simulink model "kArNa"  (R2024a)
settings: Solver=ode15s  StartTime=0.0  StopTime=721  FixedStep=0.01  MaxStep=0.5  RelTol=1e-5
PreLoadFcn:
  | %% Load parameter values:
  | 
  | load('solardata')
  | load('matincl')
  | load('trackdata3')
  | 
  | %% Parameter structures -------------------------------
  | panel = struct();
  | pipe = struct();
  | tank = struct();
  | pumps = struct();
  | 
  | %% Load parameters ------------------------------------
  | 
  | load.R = 4.5;  %Resistance. With default parameters, 4.5 Ohm is approximately optimal for maximum electrical power extraction
  | 
  | 
  | %% Solar panel parameters ------------------------------
  | 
  | % Initial temperatures [K]
  | panel.initial.Tg0 = 295; %Glass cover
  | panel.initial.Tpv0 = 295; %PV cells
  | panel.initial.Te0 = 295; %Heat exchanger
  | panel.initial.Tw0 = 295; %Water in the tank
  | panel.initial.Tb0 = 295; %Back cover
  | 
  | % Geometry
  | panel.geometry.Acell = 0.0225; %Area of a cell, [m^2]
  | panel.geometry.Ncell = 72; %Number of cells
  | 
  | % Optical properties
  | panel.optical.ng = 1.52; %Refractive index ratio glass/air
  | panel.optical.absg = 0.2; %Absorption coefficient of glass per unit length [1/m]
  | panel.optical.dg = 0.01; %Thickness of glass cover [m]
  | panel.optical.rpv = 0.15; %Reflection factor of PV cell
  | 
  | % Heat transfer properties
  | panel.heatTransfer.Ta = 295;  %Temperature of ambient air [K]
  | panel.heatTransfer.Tsky = 290;%Temperature of sky (for radiative heat transfer) [K]
  | 
  | panel.heatTransfer.Mg = 4; %Mass of glass cover [kg]
  | panel.heatTransfer.Mpv = 0.2; %Mass of one PV cell [kg]
  | panel.heatTransfer.Me = 15; %Mass of heat exchanger [kg]
  | panel.heatTransfer.Mb = 5; %Mass of back cover [kg]
  | 
  | panel.heatTransfer.Cg = 800; %Specific heat of glass [J/kg/K]
  | panel.heatTransfer.Cpv = 200; %Specific heat of PV cell [J/kg/K]
  | panel.heatTransfer.Ce = 460; %Specific heat of heat exchanger [J/kg/K]
  | panel.heatTransfer.Cb = 400; %Specific heat of back cover [J/kg/K]
  | 
  | panel.heatTransfer.epsg = 0.75; %Emissivity of glass
  | panel.heatTransfer.epspv = 0.7; %Emissivity of PV cell
  | 
  | panel.heatTransfer.hga = 10;%Free convection coefficient between glass and ambient air [W/m^2/K]
  | panel.heatTransfer.hgpv = 20; %Free convection coefficient between PV cells and glass [W/m^2/K]
  | panel.heatTransfer.hba = 10;%Free convection coefficient between back cover and ambient air [W/m^2/K]
  | 
  | panel.heatTransfer.ke = 130;%Thermal conductivity of heat exchanger [W/m/K]
  | panel.heatTransfer.Le = 0.04;%Thickness of heat exchanger [m]
  | panel.heatTransfer.kins = 0.1;%Thermal conductivity of insulation layer [W/m/K]
  | panel.heatTransfer.Lins = 0.03;%Thickness of insulation layer [m]
  | 
  | % PV cell electrical properties
  | panel.pv.Isc = 8.88; % Short-circuit current, Isc [A]
  | panel.pv.Voc = 0.62;% Open-circuit voltage, Voc [V]
  | panel.pv.Is  = 1e-6; % Diode saturation current, Is [A]
  | panel.pv.Is2 = 0; % Diode saturation current, Is2 [A]
  | panel.pv.Iph0 = 8.88;% Solar-generated current for measurements, Iph0 [A]
  | panel.pv.Ir0 = 1000;% Irradiance used for measurements, Ir0 [W/m^2]
  | panel.pv.ec = 1.5; % Quality factor, N
  | panel.pv.N2 = 2; % Quality factor, N2
  | panel.pv.Rs = 0;  % Series resistance, Rs [Ohm]
  | panel.pv.Rp = inf ; % Parallel resistance, Rp [Ohm]
  | panel.pv.TIPH1 = 0; % First order temperature coefficient for Iph, TIPH1 [1/K]
  | panel.pv.EG  = 1.11;% Energy gap, EG [eV]
  | panel.pv.TXIS1 = 3;% Temperature exponent for Is, TXIS1
  | panel.pv.TXIS2 = 3;% Temperature exponent for Is2, TXIS2
  | panel.pv.TRS1 = 0;% Temperature exponent for Rs, TRS1
  | panel.pv.TRP1 = 0;% Temperature exponent for Rp, TRP1
  | panel.pv.Tmeas = 25; % Measurement temperature [degC]
model workspace: external: MATLAB File sm_solar_tracker_parameters.m (data not in the file)
values from neighbouring files (symbols this model uses):
  matincl = [1.57079632679 1.57079632679 1.57079632679 1.57079632679 1.57079632679 1.57079632679 1.57079632679 1.57079632679 1.57079632679 1.57079632679 1.57079632679 1.57079632679 ... (721 elements, 1x721)]    [matincl.mat]
  solardata = [0 0 0 0 0 0 0 0 0 0 0 0 ... (721 elements, 1x721)]    [solardata.mat]
  trackdata3 = [3.66156931996e-23 3.03330898688e-07 9.13986174438e-07 1.77569311168e-06 2.76980746682e-06 3.72542605559e-06 4.44246757577e-06 4.72588119878e-06 4.72601258328e-06 4.79496576622e-06 5.00722746548e-06 5.38898182365e-06 ... (721 elements, 1x721)]    [trackdata3.mat]
undefined symbols (not defined in the file or in its folder): X, Y, Z
libraries: fl_lib x14, nesl_utility x11, WormAndGearConstraintLibrary x6, sm_lib x4, ee_lib x2, dspsigops x1
CloseFcn:
  | %% Close figures
  | try, close(figHandlePumpInputs), end;
  | try, close(figHandleSolarInputs), end;
  | try, close(figHandleOptics), end;
  | try, close(figHandleOutputs), end;
  | 
  | clear load
  | clear panel
  | clear pipe
  | clear pumps
  | clear tank
  | 
  | clear Absg angle demand_t demand_y E_elec E_input E_therm E_therm_source;
  | clear figHandleOptics figHandleOutputs figHandlePumpInputs figHandleSolarInputs;
  | clear internal_flow_t internal_flow_y model out Pow_elec_series Pow_input_series;
  | clear Pow_therm_series Pow_therm_source_series Reflg solar_inclination_series;
  | clear solar_inclination_t solar_inclination_y solar_irradiance_series;
  | clear solar_irradiance_t solar_irradiance_y stptime supply_t supply_y;
  | clear Tb_series Te_series Tg_series tout Tpv_series Transg Tw_series Voltank_series;
  | clear absg dg ng nga r1 r1p r1s r2 r2p r2s t1 t2 taug th2
Description:
  | Using the Worm and Gear Constraint Block - Solar Tracker
  | 
  | 
  | Copyright 2008-2019 The MathWorks, Inc.
settings Model: Creator=MathWorks  LastModifiedBy=manik
settings SolverCC: AlgebraicLoopSolver=TrustRegion
settings DataIOCC: ReturnWorkspaceOutputs=off
settings DebuggingCC: UnconnectedInputMsg=warning  UnconnectedOutputMsg=warning  UnconnectedLineMsg=warning  ArithmeticOperatorsInVariantConditions=warning
settings ModelReferenceCC: EnableRefExpFcnMdlSchedulingChecks=on
settings SFSimCC: SimUseLocalCustomCode=off  CustomCodeUndefinedFunction=UseInterfaceOnly
settings RTWCC: RTWUseLocalCustomCode=off  GPUComputeCapability=3.5
settings CodeAppCC: StateflowObjectComments=on
settings ConfigComp: CovMetricSettings=dswe
settings SimscapeCC: SimscapeNormalizeSystem=off  SimscapeNominalValues="[{\"value\":\"10\",\"unit\":\"V\"},{\"value\":\"1\",\"unit\":\"A\"},{\"value\":\"10\",\"unit\":\"N*m\"},{\"value\":\"10\",\"unit\":\"bar\"},{\"value\":\"100\",\"unit\":\"kJ/kg\"},{\"value\":\"1\",\"unit\":\"kW\"},{\"value\":\"300\",\"unit\":\"K\"},{\"value\":\"100\",\"unit\":\"cm^3/s\"},{\"value\":\"1\",\"unit\":\"kN\"},{\"value\":\"1\",\"unit\":\"g/cm^3\"},{\"value\":\"1\",\"unit\":\"l\"},{\"value\":\"1\",\"unit\":\"cm^2\"},{\"value\":\"60\",\"unit\":\"Hz\"}]"  SimscapeLogType=all  SimscapeLogSimulationStatistics=on  SimscapeLogName=simlog_sm_solar_tracker
settings DiagnosticsConfigSet: SimMechanicsUnconnectedFramePorts=none
settings ExplorerConfigSet: InternalSimMechanicsExplorerSettings="<ExplorerConfiguration><canonicalview>default</canonicalview><AnimationSetting><BasePlaybackSpeed>1.0</BasePlaybackSpeed><PlaybackSpeedFactor>256.0</PlaybackSpeedFactor></AnimationSetting><TilePanel><TileInfo><Tiles Columns=\"2\" Count=\"4\" Rows=\"2\"><Column Weight=\"0.4991\"/><Column Weight=\"0.5009\"/><Row Weight=\"0.5\"/><Row Weight=\"0.5\"/><Tile Height=\"1\" Width=\"1\" X=\"0\" Y=\"0\"/><Tile Height=\"1\" Width=\"1\" X=\"0\" Y=\"1\"/><Tile Height=\"1\" Width=\"1\" X=\"1\" Y=\"0\"/><Tile Height=\"1\" Width=\"1\" X=\"1\" Y=\"1\"/></Tiles></TileInfo><SceneInfo><SceneViewer><BGColor><R>0.60000002384185791</R><G>0.60000002384185791</G><B>0.60000002384185791</B></BGColor><Camera><DoPerspective>off</DoPerspective><Position><X>-1.59395585619392932e-09</X><Y>-1.37838790385234322</Y><Z>0.873406468711440231</Z></Position><Center><X>-1.59395585619392932e-09</X><Y>0.0359901942601611458</Y><Z>0.873406468711440231</Z></Center><Up><X>0</X><Y>-0</Y><Z>1</Z></Up><ViewLimDist>1</ViewLimDist><YLim>0.899608663916587892</YLim><XLim>1.56307005355507145</XLim></Camera></SceneViewer><SceneViewer><BGColor><R>0.60000002384185791</R><G>0.60000002384185791</G><B>0.60000002384185791</B></BGColor><Camera><DoPerspective>off</DoPerspective><Position><X>-1.59395585619392932e-09</X><Y>0.0359901942601611458</Y><Z>2.41334542087606918</Z></Position><Center><X>-1.59395585619392932e-09</X><Y>0.0359901942601611458</Y><Z>0.873406455926843073</Z></Center><Up><X>0</X><Y>1</Y><Z>-0</Z></Up><ViewLimDist>1</ViewLimDist><YLim>0.296402877697841738</YLim><XLim>0.515000000000000013</XLim></Camera></SceneViewer><SceneViewer><BGColor><R>0.60000002384185791</R><G>0.60000002384185791</G><B>0.60000002384185791</B></BGColor><Camera><DoPerspective>off</DoPerspective><Position><X>1.27256003059215272</X><Y>0.0359901942601611458</Y><Z>0.87340646871144012</Z></Position><Center><X>-1.59395585619392932e-09</X><Y>0.0359901942601611458</Y><Z>0.87340646871144012</Z></Center><Up><X>-0</X><Y>0</Y><Z>1</Z></Up><ViewLimDist>1</ViewLimDist><YLim>0.899608663916587892</YLim><XLim>1.56869260770454999</XLim></Camera></SceneViewer><SceneViewer><BGColor><R>0.60000002384185791</R><G>0.60000002384185791</G><B>0.60000002384185791</B></BGColor><Camera><DoPerspective>off</DoPerspective><Position><X>0.866331353225705314</X><Y>-0.741331845233251241</Y><Z>1.79757748242861348</Z></Position><Center><X>0.0384713109530606112</X><Y>0.0865281970393926292</Y><Z>0.969717440155970056</Z></Center><Up><X>-0.408248290463863073</X><Y>0.408248290463863073</Y><Z>0.816496580927726145</Z></Up><ViewLimDist>1</ViewLimDist><YLim>0.91983101725578309</YLim><XLim>1.60395533633977161</XLim></Camera></SceneViewer></SceneInfo></TilePanel><MechEditorPanel><Cameras><Camera><Id>Camera1</Id><Value><Name>Slew Drive View</Name><NativeCamera><PositionKeyframeSet><Keyframe><Time>0</Time><Value><X>0.052898448769590822</X><Y>3.2815089600888423</Y><Z>1.0106868675116196</Z></Value></Keyframe></PositionKeyframeSet><CenterKeyframeSet><Keyframe><Time>0</Time><Value><X>-0.01109217435380673</X><Y>3.0487464713239714</Y><Z>0.94979470185928261</Z></Value></Keyframe></CenterKeyframeSet><UpVectorKeyframeSet><Keyframe><Time>0</Time><Value><X>-0.054323829999052796</X><Y>-0.23871114009518463</Y><Z>0.96956996296744424</Z></Value></Keyframe></UpVectorKeyframeSet></NativeCamera></Value></Camera></Cameras><GfxPanelCameraMap/><VideoCreator><PlaybackSpeedRatio>1.0</PlaybackSpeedRatio><FrameRate>30</FrameRate><VideoFormat>Motion JPEG AVI</VideoFormat><FrameSize>auto</FrameSize></VideoCreator></MechEditorPanel></ExplorerConfiguration>"

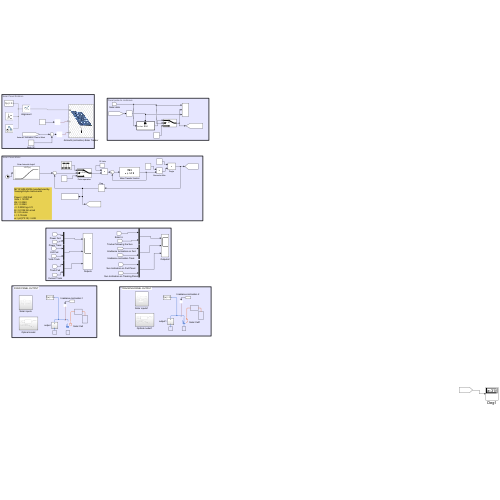
[thumbnail: Simulink's stored preview of the top-level diagram]
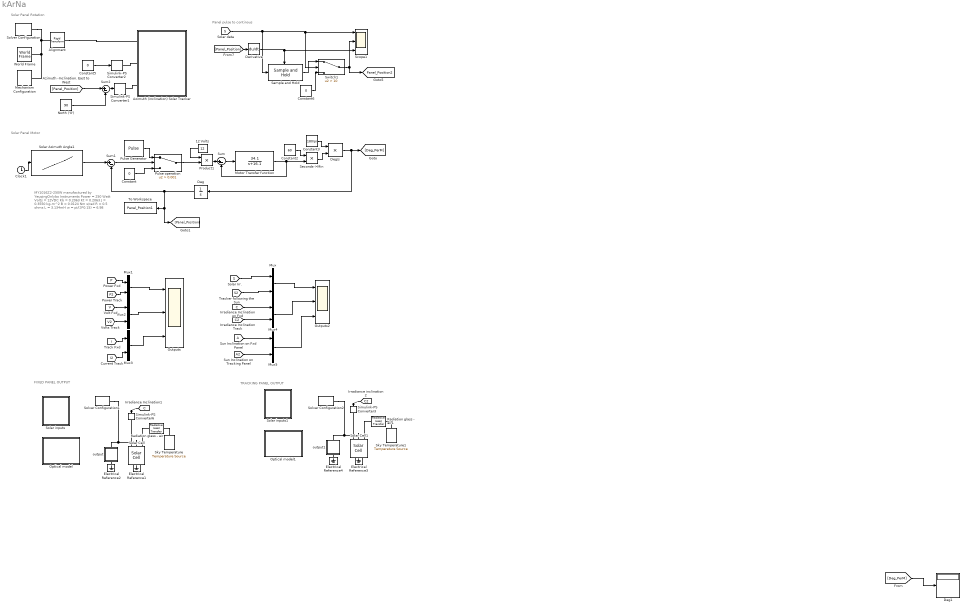
== system kArNa ==
  note: Solar Panel Motor
  note: Panel pulse to continous
  note: Solar Panel Rotation
  note: TRACKING PANEL OUTPUT
  note: FIXED PANEL OUTPUT
  note: MY1016Z2-250W manufactured by YeuqingOnlybo Instruments
      |
      | Power = 250 Watt
      | Volts = 12VDC
      | Kb = 0.2063
      | Kt = 0.2063
      | J = 0.3550 kg-m^2
      | B = 0.0124 Nm s/rad
      | R = 0.5 ohms
      | L = 3.134mH
      | w = pi/(3*0.15) = 6.98
  12 Volts : Constant  Value=12
  Alignment : sm_lib/Frames and Transforms/Rigid Transform  RotationMethod=None  FollAlignAxisA=+Z  BaseAlignAxisA=+Z  FollAlignAxisB=+Y  BaseAlignAxisB=-X  RotationStandardAxis=+Z  RotationAngle=90  RotationAngleUnits=deg  RotationArbitraryAxis=[0 0 1]  RotationSequenceAxes=FollowerAxes  RotationSequence=XYX  RotationSequenceAngles=[0 -20 0]  RotationSequenceAnglesUnits=deg  RotationMatrix=[1 0 0; 0 1 0; 0 0 1]  Quaternion=[1 0 0 0]  TranslationMethod=None  TranslationCartesianOffset=[0 0 0]  TranslationCartesianOffsetUnits=m  TranslationStandardAxis=+Z  TranslationStandardOffset=0  TranslationStandardOffsetUnits=m  TranslationROffset=0  TranslationROffsetUnits=m  TranslationThetaOffset=0  TranslationThetaOffsetUnits=deg  TranslationZOffset=0  TranslationZOffsetUnits=m
  Azimuth (inclination) Solar Tracker : Subsystem
      mask Display:
      | image(imread(fullfile(matlabroot,'toolbox','physmod','sm','smdemos','solar_tracker','images','sm_solar_tracker_solar_tracker.png')));
      | port_label('lconn',1,'B');
      | port_label('lconn',2,'y');
      | port_label('lconn',3,'p');
      | port_label('rconn',1,'w');
      | port_label('rconn',2,'t');
  Clock1 : Clock
  Constant : Constant  Value=0
  Constant2 : Constant  Value=60
  Constant3 : Constant  Value=180/pi
  Constant5 : Constant  Value=0
  Constant6 : Constant  Value=0
  Deg : Integrator
  Deg/s : Product
  Deg1 : Display
  Derivative : Derivative
  Electrical Reference{1..4} (4 alike) : fl_lib/Electrical/Electrical Elements/Electrical Reference
  Mechanism Configuration : sm_lib/Utilities/Mechanism Configuration  UniformGravity=Constant  GravityVector=[0 0 -9.80665]  GravityVectorUnits=m/s^2  LinearizationDelta=0.001  JointModeTransitionNonlinearIterations=2
  Motor Transfer function : TransferFcn  Numerator=34.1  Denominator=[1 16.1]
  Mux{,1..5} (6 alike) : Mux  Inputs=2
  North ('0') : Constant  Value=90
  Optical model : Subsystem
  Optical model1 : Subsystem
  Outputs : Scope  NumInputPorts=3
  Outputs2 : Scope  NumInputPorts=3
  Product1 : Product
  Pulse Generator : DiscretePulseGenerator  SampleTime=0.01
  Pulse operation : Switch  Criteria=u2 > Threshold  Threshold=0.001  SaturateOnIntegerOverflow=off  InputSameDT=off
  Radiation glass - air : fl_lib/Thermal/Thermal Elements/Radiative Heat Transfer  area=72*0.0225 m^2  rad_tr_coeff=5.670367e-8*0.75 W/(m^2*K^4)  T_specify=off  T_priority=None  T=0 K  T_nominal_specify=off  T_nominal_value=1  T_nominal_unit=K  Q_specify=off  Q_priority=None  Q=0 W  Q_nominal_specify=off  Q_nominal_value=1  Q_nominal_unit=W
      settings: InternalSimscapePortConfiguration="{\"Bottom\":[],\"Left\":[{\"id\":\"A\",\"label\":\"A\",\"type\":\"foundation.thermal.thermal\"}],\"Right\":[{\"id\":\"B\",\"label\":\"B\",\"type\":\"foundation.thermal.thermal\"}],\"Top\":[]}"
  Radiation glass - air1 : fl_lib/Thermal/Thermal Elements/Radiative Heat Transfer  area=72*0.0225 m^2  rad_tr_coeff=5.670367e-8*0.75 W/(m^2*K^4)  T_specify=off  T_priority=None  T=0 K  T_nominal_specify=off  T_nominal_value=1  T_nominal_unit=K  Q_specify=off  Q_priority=None  Q=0 W  Q_nominal_specify=off  Q_nominal_value=1  Q_nominal_unit=W
      settings: InternalSimscapePortConfiguration="{\"Bottom\":[],\"Left\":[{\"id\":\"A\",\"label\":\"A\",\"type\":\"foundation.thermal.thermal\"}],\"Right\":[{\"id\":\"B\",\"label\":\"B\",\"type\":\"foundation.thermal.thermal\"}],\"Top\":[]}"
  Sample and Hold : dspsigops/Sample and Hold  trig=Either edge  initCond=0  latchinput=on
  Scope1 : Scope  NumInputPorts=3
  Seconds->Min : Product
  Simulink-PS Converter1 : nesl_utility/Simulink-PS Converter  PhysicalDomain=network_engine_domain  SubClassName=ps_input  LeftPortType=input  RightPortType=output  PseudoPeriodic=off  Frequencies=[]  NoiseDistribution=none  NoiseParameters=[]  Unit=deg  AffineConversion=off  FilteringAndDerivatives=filter  SimscapeFilterOrder=2  InputFilterTimeConstant=0.2  UdotUserProvided=1
  Simulink-PS Converter2 : nesl_utility/Simulink-PS Converter  PhysicalDomain=network_engine_domain  SubClassName=ps_input  LeftPortType=input  RightPortType=output  PseudoPeriodic=off  Frequencies=[]  NoiseDistribution=none  NoiseParameters=[]  Unit=deg  AffineConversion=off  FilteringAndDerivatives=filter  SimscapeFilterOrder=2  InputFilterTimeConstant=0.2  UdotUserProvided=1
  Simulink-PS Converter3 : nesl_utility/Simulink-PS Converter  PhysicalDomain=network_engine_domain  SubClassName=ps_input  LeftPortType=input  RightPortType=output  PseudoPeriodic=off  Frequencies=[]  NoiseDistribution=none  NoiseParameters=[]  Unit=1  AffineConversion=off  FilteringAndDerivatives=provide  SimscapeFilterOrder=1  InputFilterTimeConstant=0.001  UdotUserProvided=0
  Simulink-PS Converter6 : nesl_utility/Simulink-PS Converter  PhysicalDomain=network_engine_domain  SubClassName=ps_input  LeftPortType=input  RightPortType=output  PseudoPeriodic=off  Frequencies=[]  NoiseDistribution=none  NoiseParameters=[]  Unit=1  AffineConversion=off  FilteringAndDerivatives=provide  SimscapeFilterOrder=1  InputFilterTimeConstant=0.001  UdotUserProvided=0
  Sky Temperature : fl_lib/Thermal/Thermal Sources/Temperature Source  temperature=290 K
  Sky Temperature1 : fl_lib/Thermal/Thermal Sources/Temperature Source  temperature=290 K
  Solar Azimuth Angle1 : Lookup_n-D  NumberOfTableDimensions=1  BreakpointsForDimension1=1:length(trackdata3)  Table=trackdata3  InternalRulePriority=Speed  RndMeth=Simplest
  Solar Cell : ee_lib/Sources/Solar Cell  prm=3  Isc=8.88 A  Voc=0.62 V  Is=1e-6 A  Is2=0 A  Iph=7.34 A  Ir0=1000 W/m^2  ec=1.5  N2=2  Rs=0 Ohm  Rp=inf Ohm  N_series=72  N_parallel=1  TIPH1=0 1/K  EG=1.11 eV  TXIS1=3  TXIS2=3  TRS1=0  TRP1=0  Tmeas=25 degC  TFIXED=25 degC  thermal_mass=0.2*200 J/K  initial_temperature=295 K
      settings: InternalSimscapePortConfiguration="{\"Bottom\":[],\"Left\":[{\"id\":\"Ir\",\"label\":\"Ir\",\"type\":\"input\"},{\"id\":\"p\",\"label\":\"+\",\"type\":\"foundation.electrical.electrical\"},{\"id\":\"H\",\"label\":\"H\",\"type\":\"foundation.thermal.thermal\"}],\"Right\":[{\"id\":\"n\",\"label\":\"-\",\"type\":\"foundation.electrical.electrical\"}],\"Top\":[]}"
  Solar Cell1 : ee_lib/Sources/Solar Cell  prm=3  Isc=8.88 A  Voc=0.62 V  Is=1e-6 A  Is2=0 A  Iph=7.34 A  Ir0=1000 W/m^2  ec=1.5  N2=2  Rs=0 Ohm  Rp=inf Ohm  N_series=72  N_parallel=1  TIPH1=0 1/K  EG=1.11 eV  TXIS1=3  TXIS2=3  TRS1=0  TRP1=0  Tmeas=25 degC  TFIXED=25 degC  thermal_mass=0.2*200 J/K  initial_temperature=295 K
      settings: InternalSimscapePortConfiguration="{\"Bottom\":[],\"Left\":[{\"id\":\"Ir\",\"label\":\"Ir\",\"type\":\"input\"},{\"id\":\"p\",\"label\":\"+\",\"type\":\"foundation.electrical.electrical\"},{\"id\":\"H\",\"label\":\"H\",\"type\":\"foundation.thermal.thermal\"}],\"Right\":[{\"id\":\"n\",\"label\":\"-\",\"type\":\"foundation.electrical.electrical\"}],\"Top\":[]}"
  Solar inputs : Subsystem
  Solar inputs1 : Subsystem
  Solver Configuration : nesl_utility/Solver Configuration  PhysicalDomain=network_engine_domain  SubClassName=solver  LeftPortType=input  RightPortType=generic  Tones=[]  Harmonics=[]  SimulateNoise=off  Profile=off  UseLocalSampling=off  EnableSwitchedLinearOptims=on  FrequencyDomain=off  UseCCode=off  RelTol=0.001  AbsTol=1e-06  MinStep=1e-09  ToWorkspace=off  RevertToSquareIcSolve=off  NumHomotopyIterations=100  PhasorMode=off  PhasorModeNumHarmonics=1  ConsistencySolver=NEWTON_FTOL  IndexReductionMethod=DerivativeReplacement  DoDC=off  ResidualTolerance=1e-09  ConsistencyTolSource=GLOBAL  ConsistencyAbsTol=0.001  ConsistencyRelTol=0.001  ConsistencyTolFactor=0.001  UseLocalSolver=on  LocalSolverChoice=NE_BACKWARD_EULER_ADVANCER  ResolveIndetEquations=on  FunctionEvalNumThread=1  LocalSolverSampleTime=0.1  DoFixedCost=on  MaxNonlinIter=3  MaxModeIter=2  ComputeImpulses=off  ImpulseIterations=2  LinearAlgebra=Sparse  LinearAlgebraNumThread=0  EquationFormulation=NE_TIME_EF  DelaysMemoryBudget=1024  AutomaticFiltering=on  FilteringTimeConstant=0.001  PartitionStorageMethod=AS_NEEDED  PartitionMemoryBudget=1024  PartitionMethod=FAST  MultibodyUseLocalSolver=off  MultibodyLocalSolverChoice=ODE1  MultibodyLocalSolverSampleTime=0.001
  Solver Configuration1 : nesl_utility/Solver Configuration  PhysicalDomain=network_engine_domain  SubClassName=solver  LeftPortType=input  RightPortType=generic  Tones=[]  Harmonics=[]  SimulateNoise=off  Profile=off  UseLocalSampling=off  EnableSwitchedLinearOptims=on  FrequencyDomain=off  UseCCode=off  RelTol=0.001  AbsTol=1e-06  MinStep=1e-09  ToWorkspace=off  RevertToSquareIcSolve=off  NumHomotopyIterations=100  PhasorMode=off  PhasorModeNumHarmonics=1  ConsistencySolver=NEWTON_FTOL  IndexReductionMethod=DerivativeReplacement  DoDC=off  ResidualTolerance=1e-09  ConsistencyTolSource=GLOBAL  ConsistencyAbsTol=0.001  ConsistencyRelTol=0.001  ConsistencyTolFactor=0.001  UseLocalSolver=on  LocalSolverChoice=NE_BACKWARD_EULER_ADVANCER  ResolveIndetEquations=on  FunctionEvalNumThread=1  LocalSolverSampleTime=0.1  DoFixedCost=on  MaxNonlinIter=3  MaxModeIter=2  ComputeImpulses=off  ImpulseIterations=2  LinearAlgebra=auto  LinearAlgebraNumThread=0  EquationFormulation=NE_TIME_EF  DelaysMemoryBudget=1024  AutomaticFiltering=on  FilteringTimeConstant=0.001  PartitionStorageMethod=AS_NEEDED  PartitionMemoryBudget=1024  PartitionMethod=FAST  MultibodyUseLocalSolver=off  MultibodyLocalSolverChoice=ODE1  MultibodyLocalSolverSampleTime=0.001
  Solver Configuration2 : nesl_utility/Solver Configuration  PhysicalDomain=network_engine_domain  SubClassName=solver  LeftPortType=input  RightPortType=generic  Tones=[]  Harmonics=[]  SimulateNoise=off  Profile=off  UseLocalSampling=off  EnableSwitchedLinearOptims=on  FrequencyDomain=off  UseCCode=off  RelTol=0.001  AbsTol=1e-06  MinStep=1e-09  ToWorkspace=off  RevertToSquareIcSolve=off  NumHomotopyIterations=100  PhasorMode=off  PhasorModeNumHarmonics=1  ConsistencySolver=NEWTON_FTOL  IndexReductionMethod=DerivativeReplacement  DoDC=off  ResidualTolerance=1e-09  ConsistencyTolSource=GLOBAL  ConsistencyAbsTol=0.001  ConsistencyRelTol=0.001  ConsistencyTolFactor=0.001  UseLocalSolver=on  LocalSolverChoice=NE_BACKWARD_EULER_ADVANCER  ResolveIndetEquations=on  FunctionEvalNumThread=1  LocalSolverSampleTime=0.1  DoFixedCost=on  MaxNonlinIter=3  MaxModeIter=2  ComputeImpulses=off  ImpulseIterations=2  LinearAlgebra=auto  LinearAlgebraNumThread=0  EquationFormulation=NE_TIME_EF  DelaysMemoryBudget=1024  AutomaticFiltering=on  FilteringTimeConstant=0.001  PartitionStorageMethod=AS_NEEDED  PartitionMemoryBudget=1024  PartitionMethod=FAST  MultibodyUseLocalSolver=off  MultibodyLocalSolverChoice=ODE1  MultibodyLocalSolverSampleTime=0.001
  Sum : Sum  Inputs=|+-
  Sum1 : Sum  Inputs=|+-
  Sum2 : Sum  Inputs=|+-
  "Sun Inclination on Fxd Panel " : From  TagVisibility=global
  Switch1 : Switch  Criteria=u2 > Threshold  Threshold=10  SaturateOnIntegerOverflow=off  InputSameDT=off
  To Workspace : ToWorkspace  VariableName=Panel_Position1  SaveFormat=Timeseries  SampleTime=1
  World Frame : sm_lib/Frames and Transforms/World Frame
  output : Subsystem
  output1 : Subsystem
  tag scope: Panel_Position2=global
  wires:
  Constant/1 -> Pulse operation/3
  12 Volts/1 -> Product1/1
  [Deg_PerM] -> Deg1/1
  Constant2/1 -> Seconds->Min/1
  Solar Azimuth Angle1/1 -> Sum1/1
  Pulse Generator/1 -> Pulse operation/1
  Sum/1 -> Motor Transfer function/1
  Motor Transfer function/1 -> Seconds->Min/2, Sum/2
  Seconds->Min/1 -> Deg/s/2
  Constant3/1 -> Deg/s/1
  Deg/s/1 -> [Deg_PerM], Deg/1
  Product1/1 -> Sum/1
  Pulse operation/1 -> Product1/2
  Clock1/1 -> Solar Azimuth Angle1/1
  Deg/1 -> [Panel_Position], To Workspace/1, Sum1/2
  Constant5/1 -> Simulink-PS Converter2/1
  [Panel_Position] -> Sum2/1
  North ('0')/1 -> Sum2/2
  Sum2/1 -> Simulink-PS Converter1/1
  [S] -> Sample and Hold/1, Switch1/2, Scope1/1
  [Panel_Position] -> Derivative/1
  Derivative/1 -> Sample and Hold/Trigger, Scope1/3
  Constant6/1 -> Switch1/3
  Switch1/1 -> [Panel_Position2], Scope1/2
  Sample and Hold/1 -> Switch1/1
  [C] -> Simulink-PS Converter6/1
  [S] -> Mux/1
  Mux/1 -> Outputs2/1
  [C2] -> Simulink-PS Converter3/1
  [P] -> Mux1/1
  [P2] -> Mux1/2
  Mux1/1 -> Outputs/1
  [V] -> Mux2/1
  [I] -> Mux3/1
  [I2] -> Mux3/2
  [V2] -> Mux2/2
  Mux2/1 -> Outputs/2
  Mux3/1 -> Outputs/3
  "Sun Inclination on Fxd Panel "/1 -> Mux5/1
  [A2] -> Mux5/2
  Mux4/1 -> Outputs2/2
  Mux5/1 -> Outputs2/3
  [S2] -> Mux/2
  [C] -> Mux4/1
  [C2] -> Mux4/2
  Sum1/1 -> Pulse operation/2
  connections:
  World Frame/RConn1 -- Solver Configuration/RConn1 -- Alignment/LConn1 -- Mechanism Configuration/RConn1
  Alignment/RConn1 -- Azimuth (inclination) Solar Tracker/LConn1
  Azimuth (inclination) Solar Tracker/LConn3 -- Simulink-PS Converter1/RConn1
  Azimuth (inclination) Solar Tracker/LConn2 -- Simulink-PS Converter2/RConn1
  Solver Configuration1/RConn1 -- output/RConn1 -- Solar Cell/LConn2
  Solar Cell/LConn3 -- Radiation glass - air/LConn1
  Solar Cell/RConn1 -- Electrical Reference1/LConn1
  output/LConn1 -- Electrical Reference2/LConn1
  Solar Cell/LConn1 -- Simulink-PS Converter6/RConn1
  Radiation glass - air/RConn1 -- Sky Temperature/LConn1
  Solar Cell1/LConn2 -- Solver Configuration2/RConn1 -- output1/RConn1
  Solar Cell1/LConn3 -- Radiation glass - air1/LConn1
  Radiation glass - air1/RConn1 -- Sky Temperature1/LConn1
  Solar Cell1/RConn1 -- Electrical Reference3/LConn1
  output1/LConn1 -- Electrical Reference4/LConn1
  Solar Cell1/LConn1 -- Simulink-PS Converter3/RConn1

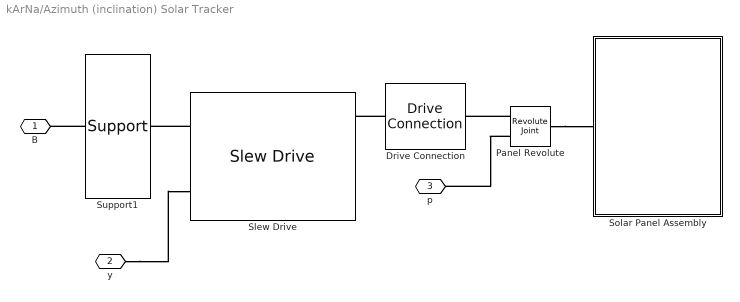
== system kArNa/Azimuth (inclination) Solar Tracker ==
  Drive Connection : WormAndGearConstraintLibrary/Drive Connection  connRadius=0.05  connThickness=0.005  connLength=0.03  bracketWidth=0.1  bracketThickness=0.15  holeRadius=0.02  holeOffset=0.06  baseThickness=0.01  rho=2700  color=[0.5,0.5,0.5]
      settings: LibrarySourceBlock=sm_solar_tracker_lib/Drive Connection
  Panel Revolute : sm_lib/Joints/Revolute Joint  JointMode=Normal  CompositeWrenchDir=FollowerOnBase  CompositeWrenchFrame=BaseFrame  SenseConstraintForce=off  SenseConstraintTorque=off  SenseTotalForce=off  SenseTotalTorque=off  PositionTargetSpecify=on  PositionTargetPriority=High  PositionTargetValue=-60  PositionTargetValueUnits=deg  VelocityTargetSpecify=off  VelocityTargetPriority=High  VelocityTargetValue=0  VelocityTargetValueUnits=deg/s  EquilibriumPosition=0  EquilibriumPositionUnits=deg  SpringStiffness=0  SpringStiffnessUnits=N*m/deg  DampingCoefficient=0  DampingCoefficientUnits=N*m/(deg/s)  LowerLimitSpecify=off  LowerLimitBound=-90  LowerLimitBoundUnits=deg  LowerLimitStiffness=1e4  LowerLimitStiffnessUnits=N*m/deg  LowerLimitDamping=10  LowerLimitDampingUnits=N*m/(deg/s)  LowerLimitTransitionRegionWidth=0.1  LowerLimitTransitionRegionWidthUnits=deg  UpperLimitSpecify=off  UpperLimitBound=90  UpperLimitBoundUnits=deg  UpperLimitStiffness=1e4  UpperLimitStiffnessUnits=N*m/deg  UpperLimitDamping=10  UpperLimitDampingUnits=N*m/(deg/s)  UpperLimitTransitionRegionWidth=0.1  UpperLimitTransitionRegionWidthUnits=deg  TorqueActuationMode=ComputedTorque  MotionActuationMode=InputMotion  SensePosition=off  SenseVelocity=off  SenseAcceleration=off  SenseTorqueForce=off  SenseLowerLimitTorqueForce=off  SenseUpperLimitTorqueForce=off
  Slew Drive : WormAndGearConstraintLibrary/Slew Drive  wormLeadAngle=10  wormLength=0.17  gearOuterRadius=0.1  gearInnerRadius=0.03  gearExposedRadius=0.06  ratio=50  housingThickness=0.005  bWormRevolute=1e-06  wormRho=7800  gearRho=7800  housingRho=2700  wormColor=[0.7,0.7,0.7]  gearColor=[0.6,0.6,0.6]  housingColor=[0.1,0.6,1]  housingOpacity=0.3
      settings: LibrarySourceBlock=sm_solar_tracker_lib/Slew Drive
  Solar Panel Assembly : Subsystem
      mask Display:
      | image(fullfile('WormAndGearConstraintSupport','Images','SolarPanel.png'));
      | port_label('lconn',1,'H');
  Support1 : WormAndGearConstraintLibrary/Support  columnRadius=0.05  columnThickness=0.005  columnHeight=0.9  baseWidth=0.2  baseThickness=0.02  rho=2700  color=[0.5,0.5,0.5]
      settings: LibrarySourceBlock=sm_solar_tracker_lib/Support
  B : PMIOPort  Side=Left
  y : PMIOPort  Port=2  Side=Left
  p : PMIOPort  Port=3  Side=Left
  connections:
  Support1/LConn1 -- B/RConn1
  Slew Drive/LConn1 -- Support1/RConn1
  Drive Connection/LConn1 -- Slew Drive/RConn1
  Panel Revolute/LConn1 -- Drive Connection/RConn1
  y/RConn1 -- Slew Drive/LConn2
  Panel Revolute/LConn2 -- p/RConn1
  Panel Revolute/RConn1 -- Solar Panel Assembly/LConn1

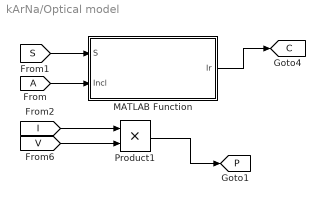
== system kArNa/Optical model ==
  From : From  TagVisibility=global
  MATLAB Function : MATLAB Function  TreatAsAtomicUnit=on
  Product1 : Product
  tag scope: C=global, P=global
  wires:
  MATLAB Function/1(Ir) -> [C]
  Product1/1 -> [P]
  [I] -> Product1/1
  [V] -> Product1/2
  From/1 -> MATLAB Function/2(Incl)
  [S] -> MATLAB Function/1(S)

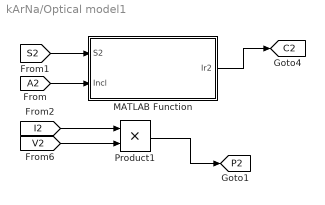
== system kArNa/Optical model1 ==
  MATLAB Function : MATLAB Function  TreatAsAtomicUnit=on
  Product1 : Product
  tag scope: C2=global, P2=global
  wires:
  MATLAB Function/1(Ir2) -> [C2]
  Product1/1 -> [P2]
  [I2] -> Product1/1
  [V2] -> Product1/2
  [A2] -> MATLAB Function/2(Incl)
  [S2] -> MATLAB Function/1(S2)

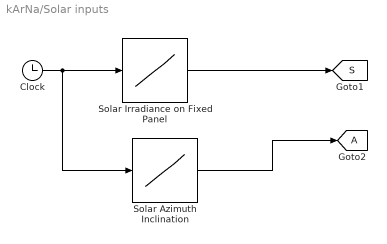
== system kArNa/Solar inputs ==
  Clock : Clock
  Goto2 : Goto  TagVisibility=global
  Solar Azimuth Inclination : Lookup_n-D  NumberOfTableDimensions=1  BreakpointsForDimension1=1:721  Table=matincl  InternalRulePriority=Speed  RndMeth=Simplest
  Solar Irradiance on Fixed Panel : Lookup_n-D  NumberOfTableDimensions=1  BreakpointsForDimension1=1:length(solardata)  Table=solardata  InternalRulePriority=Speed  RndMeth=Simplest
  tag scope: S=global
  wires:
  Solar Irradiance on Fixed Panel/1 -> [S]
  Solar Azimuth Inclination/1 -> Goto2/1
  Clock/1 -> Solar Azimuth Inclination/1, Solar Irradiance on Fixed Panel/1

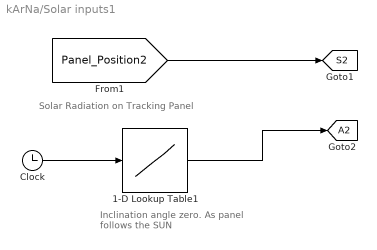
== system kArNa/Solar inputs1 ==
  note: Inclination angle zero.
      | As panel follows the SUN
  note: Solar Radiation on Tracking Panel
  1-D Lookup Table1 : Lookup_n-D  NumberOfTableDimensions=1  BreakpointsForDimension1=1:721  Table=zeros(1, 721)  InternalRulePriority=Speed  RndMeth=Simplest
  Clock : Clock
  tag scope: A2=global, S2=global
  wires:
  [Panel_Position2] -> [S2]
  1-D Lookup Table1/1 -> [A2]
  Clock/1 -> 1-D Lookup Table1/1

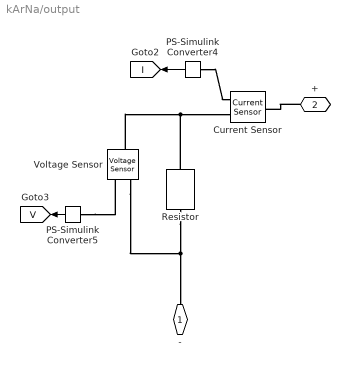
== system kArNa/output ==
  Current Sensor : fl_lib/Electrical/Electrical Sensors/Current Sensor
  PS-Simulink Converter4 : nesl_utility/PS-Simulink Converter  PhysicalDomain=network_engine_domain  SubClassName=ps_output  LeftPortType=input  RightPortType=output  PseudoPeriodic=off  Frequencies=[]  VectorFormat=1-D array  Unit=1  AffineConversion=off
  PS-Simulink Converter5 : nesl_utility/PS-Simulink Converter  PhysicalDomain=network_engine_domain  SubClassName=ps_output  LeftPortType=input  RightPortType=output  PseudoPeriodic=off  Frequencies=[]  VectorFormat=1-D array  Unit=1  AffineConversion=off
  Resistor : fl_lib/Electrical/Electrical Elements/Resistor  R=4.50 Ohm  i_specify=off  i_priority=None  i=0 A  i_nominal_specify=off  i_nominal_value=1  i_nominal_unit=A  v_specify=off  v_priority=None  v=0 V  v_nominal_specify=off  v_nominal_value=1  v_nominal_unit=V
  Voltage Sensor : fl_lib/Electrical/Electrical Sensors/Voltage Sensor
  - : PMIOPort  Side=Left
  + : PMIOPort  Port=2  Side=Right
  tag scope: I=global, V=global
  wires:
  PS-Simulink Converter4/1 -> [I]
  PS-Simulink Converter5/1 -> [V]
  connections:
  +/RConn1 -- Current Sensor/LConn1
  PS-Simulink Converter5/LConn1 -- Voltage Sensor/RConn1
  PS-Simulink Converter4/LConn1 -- Current Sensor/RConn1
  Voltage Sensor/LConn1 -- Resistor/LConn1 -- Current Sensor/RConn2
  Resistor/RConn1 -- Voltage Sensor/RConn2 -- -/RConn1

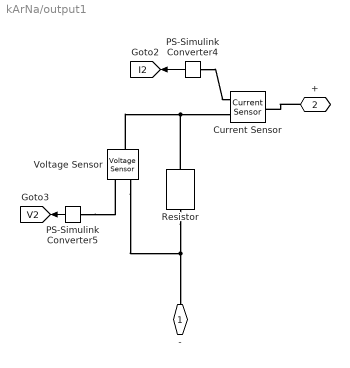
== system kArNa/output1 ==
  Current Sensor : fl_lib/Electrical/Electrical Sensors/Current Sensor
  PS-Simulink Converter4 : nesl_utility/PS-Simulink Converter  PhysicalDomain=network_engine_domain  SubClassName=ps_output  LeftPortType=input  RightPortType=output  PseudoPeriodic=off  Frequencies=[]  VectorFormat=1-D array  Unit=1  AffineConversion=off
  PS-Simulink Converter5 : nesl_utility/PS-Simulink Converter  PhysicalDomain=network_engine_domain  SubClassName=ps_output  LeftPortType=input  RightPortType=output  PseudoPeriodic=off  Frequencies=[]  VectorFormat=1-D array  Unit=1  AffineConversion=off
  Resistor : fl_lib/Electrical/Electrical Elements/Resistor  R=4.50 Ohm  i_specify=off  i_priority=None  i=0 A  i_nominal_specify=off  i_nominal_value=1  i_nominal_unit=A  v_specify=off  v_priority=None  v=0 V  v_nominal_specify=off  v_nominal_value=1  v_nominal_unit=V
  Voltage Sensor : fl_lib/Electrical/Electrical Sensors/Voltage Sensor
  - : PMIOPort  Side=Left
  + : PMIOPort  Port=2  Side=Right
  tag scope: I2=global, V2=global
  wires:
  PS-Simulink Converter4/1 -> [I2]
  PS-Simulink Converter5/1 -> [V2]
  connections:
  +/RConn1 -- Current Sensor/LConn1
  PS-Simulink Converter5/LConn1 -- Voltage Sensor/RConn1
  PS-Simulink Converter4/LConn1 -- Current Sensor/RConn1
  Voltage Sensor/LConn1 -- Resistor/LConn1 -- Current Sensor/RConn2
  Resistor/RConn1 -- Voltage Sensor/RConn2 -- -/RConn1

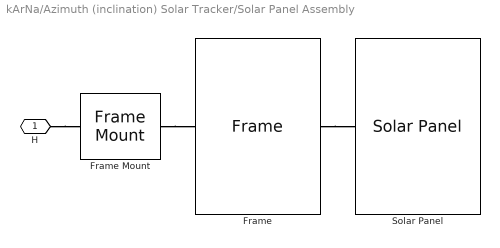
== system kArNa/Azimuth (inclination) Solar Tracker/Solar Panel Assembly ==
  Frame : WormAndGearConstraintLibrary/Frame  width=1  height=1.4  depth=0.1  beamWidth=0.05  beamThickness=0.01  frameWidth=0.02  frameThickness=0.005  rho=2700  beamColor=[0.5,0.5,0.5]  frameColor=[0.7,0.7,0.7]
      settings: LibrarySourceBlock=sm_solar_tracker_lib/Frame
  Frame Mount : WormAndGearConstraintLibrary/Frame Mount  bracketWidth=0.1  bracketThickness=0.01  bracketOffset=0.18  holeRadius=0.02  holeOffset=0.06  baseThickness=0.01  rho=2700  mountColor=[0.5,0.5,0.5]  pinColor=[0.3,0.3,0.3]
      settings: LibrarySourceBlock=sm_solar_tracker_lib/Frame Mount
  Solar Panel : WormAndGearConstraintLibrary/Solar Panel  width=1  height=1.4  frameWidth=0.02  frameDepth=0.01  cellsRho=100  frameRho=950  cellsColor=[0,0,0.5]  frameColor=[0.9,0.9,0.9]
      settings: LibrarySourceBlock=sm_solar_tracker_lib/Solar Panel
  H : PMIOPort  Side=Left
  connections:
  Frame/RConn1 -- Solar Panel/LConn1
  Frame Mount/LConn1 -- Frame/LConn1
  H/RConn1 -- Frame Mount/RConn1

== matlab function kArNa/Optical model1/MATLAB Function ==
  data: S2 input; Ir2 output; Incl input
function Ir2 = optics2(S2, Incl)
    
    %This function computes the reflection, absorption and transmission in
    %the glass to compute the irradiation to the PV cells, the heat absorbed 
    %in the glass and the radiation power absorbed in the PV cells,
    %it is based on Fresnel's laws, depending on the incident angle
    
    Ncell =  72;
    Acell =  0.0225;
    ng = 1.52;
    absg = 0.2;
    dg = 0.01;
    rpv = 0.15;
   

    % Fresnel equations 1st boundary
    r1p =  ( ng^2*cos(Incl) - sqrt(ng^2 - sin(Incl)^2) )^2/( ng^2*cos(Incl) + sqrt( ng^2 - sin(Incl)^2 ) )^2; %P polarization
    r1s =  ( cos(Incl) - sqrt(ng^2 - sin(Incl)^2) )^2/( cos(Incl) + sqrt( ng^2 - sin(Incl)^2 ) )^2; %S polarization
    r1 = 0.5*(r1p + r1s); %Effective reflectance
    t1 = 1-r1;

    nga = 1/ng; %refractive index glass -> air
    th2 = asin(sin(Incl)/ng);  %Snell's law to compute angle of incidence on 2nd boundary

    % Fresnel equations 2nd boundary
    r2p = ( nga^2*cos(th2) - sqrt(nga^2 - sin(th2)^2) )^2/( nga^2*cos(th2) + sqrt( nga^2 - sin(th2)^2 ) )^2 ;
    r2s = ( cos(th2) - sqrt(nga^2 - sin(th2)^2) )^2/( cos(th2) + sqrt( nga^2 - sin(th2)^2 ) )^2 ;
    r2 = 0.5*(r2p + r2s); %Effective reflectance
    t2 = 1 - r2;

    taug = exp(-absg*dg/cos(th2)); 
    
    %Total coefficients for infinite reflections between 2 parallel boundaries
    Transg = t1*taug*t2/(1 - r1*r2*taug^2);
    Reflg = r1 + (t1^2*taug^2*r2)/(1 - r1*r2*taug^2);
    Absg = 1 - Transg - Reflg; 

    Ir2 = S2*Transg; %Irradiation to the PV cells
    heatg = Acell*Ncell*Absg*S2; %heat absorbed in the glass
    powAbspv = Acell*Ncell*Transg*(1-rpv)*S2; %radiation power absorbed by PV cells. Part of it transforms in electrical power
    
end

== matlab function kArNa/Optical model/MATLAB Function ==
  data: S input; Ir output; Incl input
function Ir = optics(S, Incl)
    
    %This function computes the reflection, absorption and transmission in
    %the glass to compute the irradiation to the PV cells, the heat absorbed 
    %in the glass and the radiation power absorbed in the PV cells,
    %it is based on Fresnel's laws, depending on the incident angle
    
    Ncell =  72;
    Acell =  0.0225;
    ng = 1.52;
    absg = 0.2;
    dg = 0.01;
    rpv = 0.15;
   

    % Fresnel equations 1st boundary
    r1p =  ( ng^2*cos(Incl) - sqrt(ng^2 - sin(Incl)^2) )^2/( ng^2*cos(Incl) + sqrt( ng^2 - sin(Incl)^2 ) )^2; %P polarization
    r1s =  ( cos(Incl) - sqrt(ng^2 - sin(Incl)^2) )^2/( cos(Incl) + sqrt( ng^2 - sin(Incl)^2 ) )^2; %S polarization
    r1 = 0.5*(r1p + r1s); %Effective reflectance
    t1 = 1-r1;

    nga = 1/ng; %refractive index glass -> air
    th2 = asin(sin(Incl)/ng);  %Snell's law to compute angle of incidence on 2nd boundary

    % Fresnel equations 2nd boundary
    r2p = ( nga^2*cos(th2) - sqrt(nga^2 - sin(th2)^2) )^2/( nga^2*cos(th2) + sqrt( nga^2 - sin(th2)^2 ) )^2 ;
    r2s = ( cos(th2) - sqrt(nga^2 - sin(th2)^2) )^2/( cos(th2) + sqrt( nga^2 - sin(th2)^2 ) )^2 ;
    r2 = 0.5*(r2p + r2s); %Effective reflectance
    t2 = 1 - r2;

    taug = exp(-absg*dg/cos(th2)); 
    
    %Total coefficients for infinite reflections between 2 parallel boundaries
    Transg = t1*taug*t2/(1 - r1*r2*taug^2);
    Reflg = r1 + (t1^2*taug^2*r2)/(1 - r1*r2*taug^2);
    Absg = 1 - Transg - Reflg; 

    Ir = S*Transg; %Irradiation to the PV cells
    heatg = Acell*Ncell*Absg*S; %heat absorbed in the glass
    powAbspv = Acell*Ncell*Transg*(1-rpv)*S; %radiation power absorbed by PV cells. Part of it transforms in electrical power
    
end
